simulink model "reaction_pendulum_mpc"  (R2021b)
settings: Solver=FixedStepDiscrete  StartTime=0.0  StopTime=80  FixedStep=h  RelTol=1e-3  EnableMultiTasking=on
PreLoadFcn:
  | warning('off','MATLAB:dispatcher:InexactMatch');
InitFcn:
  | hwinit
values from neighbouring files (symbols this model uses):
  h = 0.05    [reaction_pendulum.mat]
undefined symbols (not defined in the file or in its folder): Discrete, G_disc, K_lqr, L, Time, Ts
libraries: ctrlSharedLib x1, eeLuenbergerObserver x1
settings Model: SimulationMode=external  ExtModeTrigDuration=100000  Creator=user  LastModifiedBy=xyzhang
settings SolverCC: AlgebraicLoopSolver=TrustRegion
settings DataIOCC: SaveFormat=Array  SignalLoggingSaveFormat=ModelDataLogs  SaveOutput=off  SignalLogging=off  DSMLogging=off  SaveTime=off  ReturnWorkspaceOutputs=off
settings OptimizationCC: ExpressionDepthLimit=2147483647  LifeSpan=inf
settings DebuggingCC: UnderspecifiedInitializationDetection=Classic  MergeDetectMultiDrivingBlocksExec=none  SolverPrmCheckMsg=warning  FcnCallInpInsideContextMsg=warning  StateNameClashWarn=warning  SFUnexpectedBacktrackingDiag=warning  SFNoUnconditionalDefaultTransitionDiag=warning  SFExecutionAtInitializationDiag=none  SFMachineParentedDataDiag=warning  ArithmeticOperatorsInVariantConditions=warning
settings HardwareCC: ProdBitPerPointer=32  ProdBitPerSizeT=32  ProdBitPerPtrDiffT=32  ProdLargestAtomicFloat=None  ProdIntDivRoundTo=Undefined  ProdEndianess=Unspecified  ProdWordSize=32  ProdHWDeviceType=32-bit Generic
settings ModelReferenceCC: PropagateSignalLabelsOutOfModel=off
settings SFSimCC: SimUseLocalCustomCode=off  CustomCodeUndefinedFunction=UseInterfaceOnly
settings RTWCC: Description=rpend RTDAC/USB2 (Visual C/C++)  SystemTargetFile=rtcon_rpend_usb2.tlc  TemplateMakefile=rtcon_rpend_vc_usb2_x64.tmf  RTWUseLocalCustomCode=off
settings CodeAppCC: StateflowObjectComments=on
settings STFCustomTargetCC: ModelReferenceCompliant=off  CombineOutputUpdateFcns=on  MatFileLogging=on  GRTInterface=off  SystemTargetFile=rtcon_rpend_usb2.tlc
settings GRTTargetCC: TargetLangStandard=C89/C90 (ANSI)  ModelReferenceCompliant=off  ParMdlRefBuildCompliant=off  CompOptLevelCompliant=off  ConcurrentExecutionCompliant=off  CPPClassGenCompliant=off  UseToolchainInfoCompliant=off  ExtMode=on  ExtModeMexFile=rtcon_ext_comm
settings ConfigComp: CovMetricSettings=dw  CovSaveCumulativeToWorkspaceVar=on  CovSaveSingleToWorkspaceVar=on  CovExternalEMLEnable=off  CovSFcnEnable=off

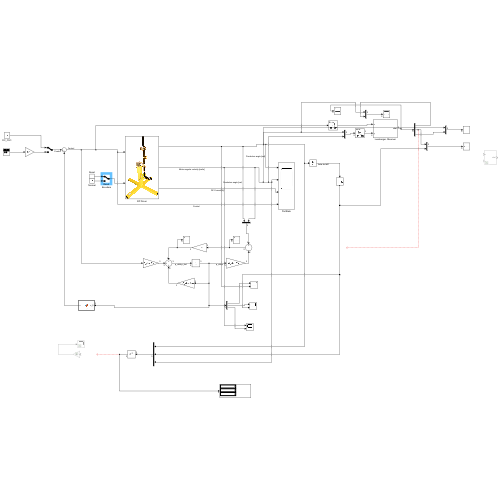
[thumbnail: Simulink's stored preview of the top-level diagram]
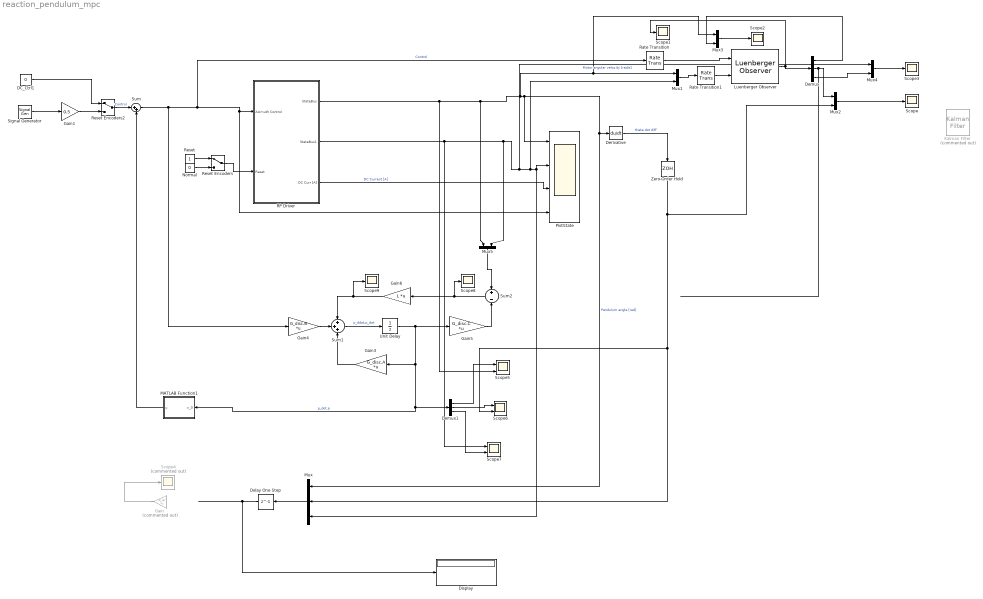
== system reaction_pendulum_mpc ==
  DC_Ctrl1 : Constant  Value=0
  Delay One Step : Delay  DelayLength=1  SampleTime=h
  Demux : Demux  Outputs=3
  Demux1 : Demux  Outputs=3
  Derivative : Derivative
  Display : Display
  Gain : Gain  Commented=on  Gain=-K_lqr  Multiplication=Matrix(K*u)
  Gain1 : Gain  Gain=0.5
  Gain3 : Gain  Gain=G_disc.A  Multiplication=Matrix(K*u)
  Gain4 : Gain  Gain=G_disc.B  Multiplication=Matrix(K*u)
  Gain5 : Gain  Gain=G_disc.C  Multiplication=Matrix(K*u)
  Gain6 : Gain  Gain=L  Multiplication=Matrix(K*u)
  Kalman Filter : ctrlSharedLib/Kalman Filter  Commented=on  TimeDomain=Discrete-Time  UseCurrentEstimator=on  ModelSource=Individual A, B, C, D matrices  ModelSourceVariable=ss(0.95,1,1,0,1)  A=G_disc.A  B=G_disc.B  C=G_disc.C  D=G_disc.D  NumberOfStates=1  NumberOfInputs=1  NumberOfOutputs=1  InitialEstimateSource=Dialog  X0=[0;0;0]  P0=10  UseK=off  UseGH=off  NumberOfProcessNoiseInputs=1  G=1  TimeInvariantG=on  H=0  TimeInvariantH=on  Q=[1e-1 0 0;0 1e4 0; 0 0 1e-1]  TimeInvariantQ=on  R=1e-1*eye(2)  TimeInvariantR=on  N=0  TimeInvariantN=on  AddInputPort=on  AddEnablePort=off  OutputEstimatedY=off  OutputP=off  Ts=h
  Luenberger Observer : eeLuenbergerObserver/Luenberger Observer  StateSpaceType=Discrete-time  Ad=G_disc.A  Bd=G_disc.B  Cd=G_disc.C  Dd=G_disc.D  A=1  B=1  C=1  D=1  ObserverDesign=Observer gain  Ld=L  DesiredEigenvalues=0  x0=[0;0;0]  Tsd=0.1  Ts=h
      settings: SourceProductBaseCode=PS
  MATLAB Function1 : MATLAB Function  TreatAsAtomicUnit=on
  Mux : Mux  Inputs=3
  Mux{1..5} (5 alike) : Mux  Inputs=2
  Normal : Constant  Value=0
  PlotState : Scope  NumInputPorts=4
  RP Driver : Subsystem
      mask Display: image(imread('rwp.JPG'))
  Rate Transition : RateTransition  OutPortSampleTime=h
  Rate Transition1 : RateTransition  OutPortSampleTime=h
  Reset : Constant
  Reset Encoders : ManualSwitch
  Reset Encoders2 : ManualSwitch
  Scope{,1..3,8..9} (6 alike) : Scope
  Scope4 : Scope  Commented=on
  Scope5 : Scope  NumInputPorts=2
  Scope6 : Scope  NumInputPorts=2
  Scope7 : Scope  NumInputPorts=2
  Signal Generator : SignalGenerator  Amplitude=0.5  Frequency=0.1
  Sum : Sum  Inputs=|++
  Sum1 : Sum  Inputs=+++
  Sum2 : Sum  Inputs=+-
  Unit Delay : UnitDelay  SampleTime=Ts  HasFrameUpgradeWarning=on
  Zero-Order Hold : ZeroOrderHold  SampleTime=-1
  wires:
  Normal/1 -> Reset Encoders/2
  Reset/1 -> Reset Encoders/1
  Reset Encoders/1 -> RP Driver/2(Reset)
  RP Driver/3(DC Curr [A]) -> PlotState/3  "DC Current [A]"
  Sum/1 -> Gain4/1, Rate Transition/1, PlotState/4, RP Driver/1(Azimuth Control)  "Control"
  DC_Ctrl1/1 -> Reset Encoders2/1
  Signal Generator/1 -> Gain1/1
  Gain1/1 -> Reset Encoders2/2
  Derivative/1 -> Zero-Order Hold/1  "theta dot diff"
  RP Driver/1(StateBus) -> Scope5/2, PlotState/1, Mux/1, Derivative/1, Mux3/1, Mux1/1, Mux5/1  "Pendulum angle [rad]"
  Mux/1 -> Delay One Step/1
  RP Driver/2(StateBus1) -> Mux5/2, Mux4/1, PlotState/2, Mux/3, Mux1/2, Scope7/1  "Motor angular velocity [rad/s]"
  Gain/1 -> Scope4/1
  Delay One Step/1 -> Display/1
  Reset Encoders2/1 -> Sum/1  "Control"
  Luenberger Observer/1 -> Demux/1, Scope1/1
  Mux2/1 -> Scope/1
  Demux/2 -> Mux2/1
  Rate Transition/1 -> Luenberger Observer/1
  Mux1/1 -> Rate Transition1/1
  Rate Transition1/1 -> Luenberger Observer/2
  Zero-Order Hold/1 -> Mux2/2, Scope6/2, Mux/2
  Mux3/1 -> Scope2/1
  Demux/1 -> Mux3/2
  Mux4/1 -> Scope3/1
  Demux/3 -> Mux4/2
  Gain4/1 -> Sum1/2
  Unit Delay/1 -> MATLAB Function1/1(x_0), Demux1/1, Gain3/1, Gain5/1  "p_dot,p"
  Sum1/1 -> Unit Delay/1  "p_ddot,p_dot"
  Sum2/1 -> Scope8/1, Gain6/1
  Gain6/1 -> Scope9/1, Sum1/1
  Gain3/1 -> Sum1/3
  Demux1/1 -> Scope5/1
  Demux1/2 -> Scope6/1
  Demux1/3 -> Scope7/2
  Mux5/1 -> Sum2/1
  Gain5/1 -> Sum2/2
  MATLAB Function1/1(u) -> Sum/2

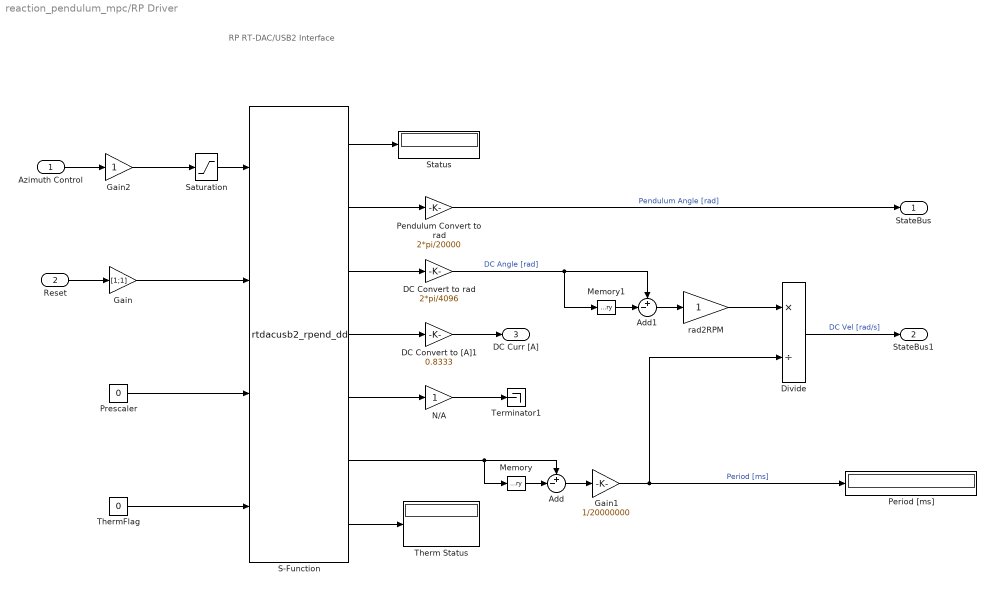
== system reaction_pendulum_mpc/RP Driver ==
  note: RP RT-DAC/USB2
      | Interface
  Azimuth Control : Inport
  Reset : Inport  Port=2
  Add : Sum  Inputs=+-|
  Add1 : Sum  Inputs=+-|
  DC Convert to [A]1 : Gain  Gain=0.8333  SaturateOnIntegerOverflow=on  OutDataTypeStr=Inherit: Same as input  ParamDataTypeStr=Inherit: Same as input
  DC Convert to rad : Gain  Gain=2*pi/4096  SaturateOnIntegerOverflow=on  OutDataTypeStr=Inherit: Same as input  ParamDataTypeStr=Inherit: Same as input
  Divide : Product  Inputs=*/
  Gain : Gain  Gain=[1;1]
  Gain1 : Gain  Gain=1/20000000
  Gain2 : Gain
  Memory : Memory
  Memory1 : Memory
  N/A : Gain  SaturateOnIntegerOverflow=on  OutDataTypeStr=Inherit: Same as input  ParamDataTypeStr=Inherit: Same as input
  Pendulum Convert to rad : Gain  Gain=2*pi/20000  SaturateOnIntegerOverflow=on  OutDataTypeStr=Inherit: Same as input  ParamDataTypeStr=Inherit: Same as input
  Period [ms] : Display
  Prescaler : Constant  Value=0
  S-Function : S-Function  FunctionName=rtdacusb2_rpend_dd  Parameters=1, h  SFunctionDeploymentMode=off  EnableBusSupport=off
  Saturation : Saturate  UpperLimit=1  LowerLimit=-1
  Status : Display
  Terminator1 : Terminator
  Therm Status : Display
  ThermFlag : Constant  Value=0
  rad2RPM : Gain  SaturateOnIntegerOverflow=on  OutDataTypeStr=Inherit: Same as input  ParamDataTypeStr=Inherit: Same as input
  StateBus : Outport  VectorParamsAs1DForOutWhenUnconnected=off
  StateBus1 : Outport  Port=2  VectorParamsAs1DForOutWhenUnconnected=off
  DC Curr [A] : Outport  Port=3  VectorParamsAs1DForOutWhenUnconnected=off
  wires:
  S-Function/7 -> Therm Status/1
  S-Function/5 -> N/A/1
  S-Function/4 -> DC Convert to [A]1/1
  ThermFlag/1 -> S-Function/4
  Prescaler/1 -> S-Function/3
  Gain/1 -> S-Function/2
  DC Convert to [A]1/1 -> DC Curr [A]/1
  Divide/1 -> StateBus1/1  "DC Vel [rad/s]"
  rad2RPM/1 -> Divide/1
  Add1/1 -> rad2RPM/1
  Memory1/1 -> Add1/2
  N/A/1 -> Terminator1/1
  S-Function/6 -> Add/1, Memory/1
  Gain2/1 -> Saturation/1
  Gain1/1 -> Period [ms]/1, Divide/2  "Period [ms]"
  Add/1 -> Gain1/1
  Memory/1 -> Add/2
  DC Convert to rad/1 -> Add1/1, Memory1/1  "DC Angle [rad]"
  S-Function/3 -> DC Convert to rad/1
  Pendulum Convert to rad/1 -> StateBus/1  "Pendulum Angle [rad]"
  S-Function/2 -> Pendulum Convert to rad/1
  S-Function/1 -> Status/1
  Saturation/1 -> S-Function/1
  Reset/1 -> Gain/1
  Azimuth Control/1 -> Gain2/1

== matlab function reaction_pendulum_mpc/MATLAB Function1 ==
  data: u output; x_0 input

function u = fcn(x_0)

G_disc.A = [1.01245621948217 0.0500306038965976 1.40121956403498e-05;
    0.498695053520506 1.00537188597042 0.000556377324148220;
    0 0 0.951367362767549]; 
G_disc.B = [-0.00374072094651530;
    -0.148158292603784;
    16.9179146743878];
G_disc.C = [1 0 0; 0 0 1];
G_disc.D = [0;0];


weight.Q =[4.5 0 0;0 3.5 0; 0 0 0.0071];   % weight on output
weight.R = 20;

weight.P = [33902.9619566707 10451.8828677435 65.3859904844755;
    10451.8828677435 3236.36403267760 20.2149858869273;
    65.3859904844755 20.2149858869273 0.149003450051045];


umin = -0.11; % 0.1 A as rated current
umax = -umin;  
dim.nx = size(G_disc.A,1); % state dimension
dim.nu = size(G_disc.B,2); % input dimension
dim.ny = size(G_disc.C,1);
dim.N = 40;

% Define prediction model + cost
[S,T] = predmodgen(G_disc,dim);

% Cost definition
Q_bar = blkdiag(kron(eye(dim.N), weight.Q), weight.P);
H = S' * Q_bar * S + kron(eye(dim.N),weight.R);   
h = S' * Q_bar * T;

% Inequality Constraints
x1_constraint = 0.25; % it is about 17 degrees
x2_constraint = 2; % 0.3/0.05 --> goes from 0.3 rad to 0 in one time step
x3_constraint = 400; % about 85 rad/sec (see datasheet)

up =[x1_constraint; x2_constraint; x3_constraint];
lb = -up;
bounds = [up; -lb];
eps = repmat(bounds, dim.N+1,1);

f = [eye(3); -eye(3)];
F = kron(eye(dim.N+1), f);
eps_1 = F*T;

A_in = F*S;  

% Equality constraints (terminal)
Ae = S(end-dim.nx+1:end,:);
be = T(end-dim.nx+1:end,:);


%% MPC

    A_in = [A_in]%; A_in_Tset*Ae];
    b_in = [eps - eps_1*x_0]%; (b_in_Tset - A_in_Tset*be*x_0 )];
    lb = umin*ones(dim.N,1);
    ub = umax*ones(dim.N,1);
    options = optimoptions('quadprog','Display','iter', "Algorithm",'active-set');
    init_val = zeros(dim.N,1)';
    u_horizon = quadprog(H, (h * x_0), A_in, b_in, [],[], lb, ub, init_val,options )
    
    u=u_horizon(1);
%% Define prediction model 

% Generation of prediction model -> Prediction matrix from initial state
function [S,T]=predmodgen(LTI,dim)

T=zeros(dim.nx*(dim.N+1),dim.nx); % nx = 4

for k=0:dim.N
    T(k*dim.nx+1:(k+1)*dim.nx,:)=LTI.A^k;
end

%Prediction matrix from input
S=zeros(dim.nx*(dim.N+1),dim.nu*(dim.N));
for k=1:dim.N
    for i=0:k-1
        S(k*dim.nx+1:(k+1)*dim.nx,i*dim.nu+1:(i+1)*dim.nu)=LTI.A^(k-1-i)*LTI.B;
    end
end

predmod.T=T;
predmod.S=S;

end
end
